simulink model "gm_pulse_detector_v4_4_vnl"  (R2017b)
settings: Solver=FixedStepDiscrete  StartTime=0.0  StopTime=SimTime  RelTol=1e-3
undefined symbols (not defined in the file or in its folder): CorrFilter, rowCorrFilter, RxSignal, threshold, WindowLen
libraries: simulink x5, dspsrcs4 x2, dsphdlfiltering x1, hdlsllib x1
settings Model: SimulationMode=accelerator  Creator=proso  LastModifiedBy=proso
settings DataIOCC: SaveOutput=off  SaveTime=off  ReturnWorkspaceOutputs=on
settings OptimizationCC: BlockReduction=off  ConditionallyExecuteInputs=off  DefaultParameterBehavior=Inlined
settings DebuggingCC: AlgebraicLoopMsg=error  InheritedTsInSrcMsg=none  SingleTaskRateTransMsg=error
settings HardwareCC: ProdBitPerPointer=32  ProdBitPerSizeT=32  ProdBitPerPtrDiffT=32  ProdLargestAtomicFloat=None  ProdIntDivRoundTo=Undefined  ProdEndianess=Unspecified  ProdWordSize=32  ProdHWDeviceType=ASIC/FPGA->ASIC/FPGA  TargetBitPerPointer=64  TargetBitPerSizeT=64  TargetBitPerPtrDiffT=64  TargetLongLongMode=on  TargetIntDivRoundTo=Zero  TargetEndianess=LittleEndian  TargetWordSize=64  TargetHWDeviceType=Custom Processor->MATLAB Host Computer  ProdEqTarget=off

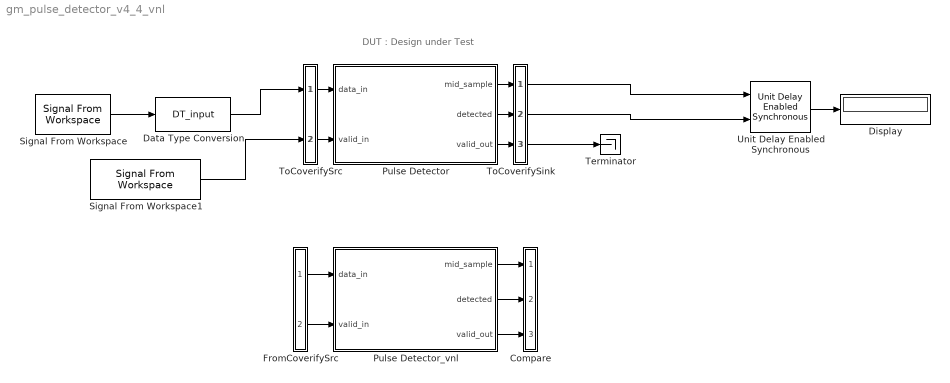
== system gm_pulse_detector_v4_4_vnl ==
  note: DUT : Design under Test
  Compare : Subsystem
      mask Display: disp('')
  Data Type Conversion : DataTypeConversion  OutDataTypeStr=DT_input
  Display : Display
  FromCoverifySrc : Subsystem
      mask Display: disp('')
  Pulse Detector : Subsystem
  Pulse Detector_vnl : Subsystem
  Signal From Workspace : dspsrcs4/Signal From Workspace  X=RxSignal  Ts=1  nsamps=1  OutputAfterFinalValue=Setting to zero  ignoreOrWarnInputAndFrameLengths=off  OutputFrames=off
  Signal From Workspace1 : dspsrcs4/Signal From Workspace  X=true(size(RxSignal))  Ts=1  nsamps=1  OutputAfterFinalValue=Setting to zero  ignoreOrWarnInputAndFrameLengths=off  OutputFrames=off
  Terminator : Terminator
  ToCoverifySink : Subsystem
      mask Display: disp('')
  ToCoverifySrc : Subsystem
      mask Display: disp('')
  Unit Delay Enabled Synchronous : hdlsllib/Discrete/Unit Delay Enabled Synchronous  InitialCondition=0.0  SampleTime=-1
      settings: SourceProductName=HDL Coder  SourceProductBaseCode=HD
  wires:
  Unit Delay Enabled Synchronous/1 -> Display/1
  Signal From Workspace/1 -> Data Type Conversion/1
  ToCoverifySrc/1(out1) -> Pulse Detector/1(data_in)
  ToCoverifySrc/2(out2) -> Pulse Detector/2(valid_in)
  Pulse Detector/1(mid_sample) -> ToCoverifySink/1(in1)
  Pulse Detector/2(detected) -> ToCoverifySink/2(in2)
  Pulse Detector/3(valid_out) -> ToCoverifySink/3(in3)
  Data Type Conversion/1 -> ToCoverifySrc/1(in1)
  Signal From Workspace1/1 -> ToCoverifySrc/2(in2)
  ToCoverifySink/1(out1) -> Unit Delay Enabled Synchronous/1
  ToCoverifySink/2(out2) -> Unit Delay Enabled Synchronous/2
  ToCoverifySink/3(out3) -> Terminator/1
  FromCoverifySrc/1(out1) -> Pulse Detector_vnl/1(data_in)
  FromCoverifySrc/2(out2) -> Pulse Detector_vnl/2(valid_in)
  Pulse Detector_vnl/1(mid_sample) -> Compare/1(in1)
  Pulse Detector_vnl/2(detected) -> Compare/2(in2)
  Pulse Detector_vnl/3(valid_out) -> Compare/3(in3)

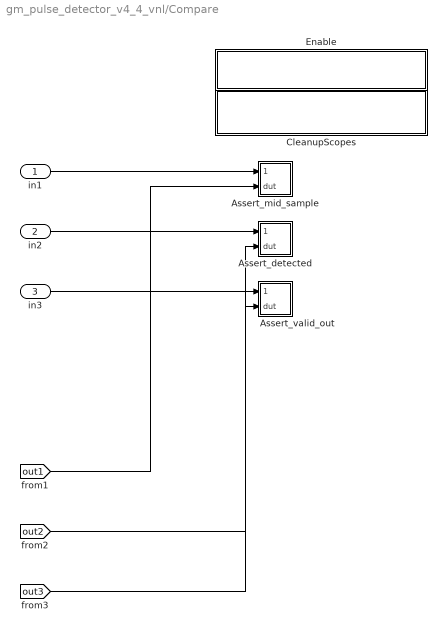
== system gm_pulse_detector_v4_4_vnl/Compare ==
  in1 : Inport
  in2 : Inport  Port=2
  in3 : Inport  Port=3
  Assert_detected : Subsystem
  Assert_mid_sample : Subsystem
  Assert_valid_out : Subsystem
  CleanupScopes : Subsystem
      settings: OpenFcn=|
      | blkName = gcb; %self block
      | idx = regexp(blkName, '/CleanupScopes$', 'once');
      | blkParent = blkName(1:idx-1);
      | blks=find_system(blkParent, 'LookUnderMasks', 'all','blocktype', 'Scope');
      | for itr = 1:length(blks)
      | 	 hScopeCfg = get_param(blks{itr},'ScopeConfiguration');
      | 	 hScopeCfg.Visible = ~ hScopeCfg.Visible;
      | end
      | drawnow;
      mask Display: fprintf(message('hdlcoder:cosim:vnl_dblclick').getString());
  Enable : Subsystem
      settings: OpenFcn=|
      | blkName = gcb;
      | idx = regexp(blkName, '/Enable$', 'once');
      | blkParent = blkName(1:idx-1);
      | blks=find_system(blkParent, 'LookUnderMasks', 'all','blocktype', 'Assertion');
      | e = get_param(blks{1}, 'Enabled');
      | if strcmp(e, 'on'), f= 'off';, else, f = 'on';, end
      | for ii=1:length(blks), set_param(blks{ii}, 'Enabled', f);, end
      | set_param(gcb, 'MaskDisplay',['fprintf(message(''hdlcoder:cosim:vnl_dblclick_assertions'',','''',upper(e),'''',').getString())']);
      mask Display: fprintf(message('hdlcoder:cosim:vnl_dblclick_assertions','OFF').getString());
  wires:
  in1/1 -> Assert_mid_sample/1(cosim)
  [out1] -> Assert_mid_sample/2(dut)
  in2/1 -> Assert_detected/1(cosim)
  [out2] -> Assert_detected/2(dut)
  in3/1 -> Assert_valid_out/1(cosim)
  [out3] -> Assert_valid_out/2(dut)

== system gm_pulse_detector_v4_4_vnl/FromCoverifySrc ==
  out1 : Outport
  out2 : Outport  Port=2
  wires:
  [in1] -> out1/1
  [in2] -> out2/1

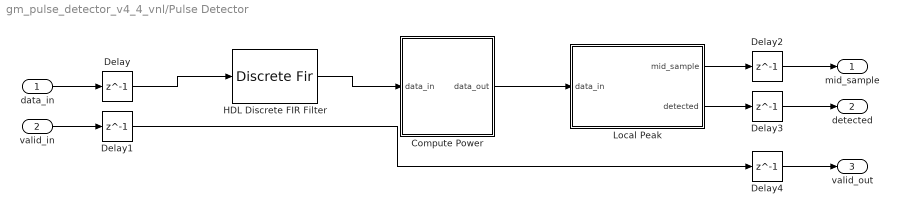
== system gm_pulse_detector_v4_4_vnl/Pulse Detector ==
  data_in : Inport  OutDataTypeStr=fixdt(1, 16, 14)  SampleTime=1
      settings: SignalType=complex
  valid_in : Inport  Port=2  OutDataTypeStr=boolean  SampleTime=1
  Compute Power : Subsystem
  Delay{,1..4} (5 alike) : Delay  DelayLength=1
  HDL Discrete FIR Filter : DiscreteFir  FilterStructure=Direct form transposed  Coefficients=CorrFilter  CoefDataTypeStr=DT_coeff
  Local Peak : Subsystem
  mid_sample : Outport
  detected : Outport  Port=2
  valid_out : Outport  Port=3
  wires:
  Local Peak/2(detected) -> Delay3/1
  Local Peak/1(mid_sample) -> Delay2/1
  HDL Discrete FIR Filter/1 -> Compute Power/1(data_in)
  Delay4/1 -> valid_out/1
  Delay3/1 -> detected/1
  Delay2/1 -> mid_sample/1
  Delay1/1 -> Delay4/1
  Delay/1 -> HDL Discrete FIR Filter/1
  Compute Power/1(data_out) -> Local Peak/1(data_in)
  valid_in/1 -> Delay1/1
  data_in/1 -> Delay/1

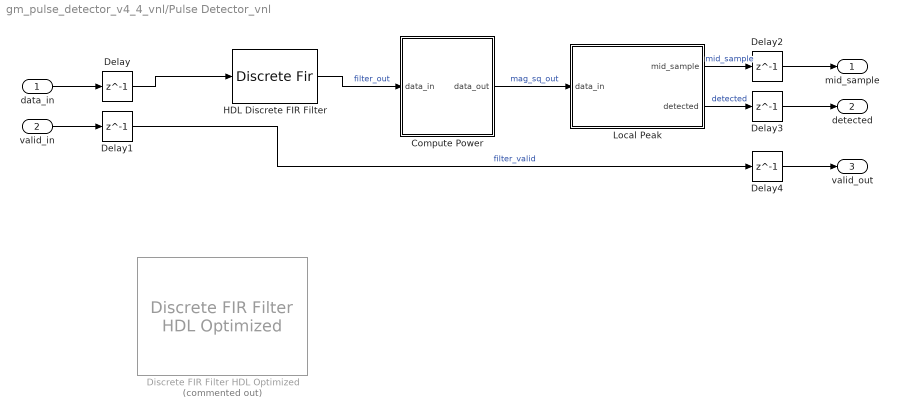
== system gm_pulse_detector_v4_4_vnl/Pulse Detector_vnl ==
  data_in : Inport
  valid_in : Inport  Port=2
  Compute Power : Subsystem
  Delay{,1..4} (5 alike) : Delay  DelayLength=1
  Discrete FIR Filter HDL Optimized : dsphdlfiltering/Discrete FIR Filter HDL Optimized  Commented=on  Numerator=real(rowCorrFilter)  Sharing=off  SharingFactor=2  SimulateUsing=Code generation  roundingMode=Floor  overflowMode=off  CoefficientsDataTypeStr=DT_coeff  CoefficientsMin=[]  CoefficientsMax=[]  OutputDataTypeStr=Inherit: Same word length as input  OutputMin=[]  OutputMax=[]  ValidInPort=on  ReadyPort=off
      settings: SourceProductName=DSP System Toolbox  SourceProductBaseCode=DS
  HDL Discrete FIR Filter : DiscreteFir  FilterStructure=Direct form transposed  Coefficients=CorrFilter  CoefDataTypeStr=DT_coeff
  Local Peak : Subsystem
  mid_sample : Outport
  detected : Outport  Port=2
  valid_out : Outport  Port=3
  wires:
  Delay4/1 -> valid_out/1
  Delay3/1 -> detected/1
  Delay2/1 -> mid_sample/1
  Delay/1 -> HDL Discrete FIR Filter/1
  Delay1/1 -> Delay4/1  "filter_valid"
  valid_in/1 -> Delay1/1
  Local Peak/2(detected) -> Delay3/1  "detected"
  data_in/1 -> Delay/1
  Local Peak/1(mid_sample) -> Delay2/1  "mid_sample"
  Compute Power/1(data_out) -> Local Peak/1(data_in)  "mag_sq_out"
  HDL Discrete FIR Filter/1 -> Compute Power/1(data_in)  "filter_out"

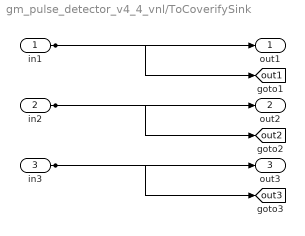
== system gm_pulse_detector_v4_4_vnl/ToCoverifySink ==
  in1 : Inport
  in2 : Inport  Port=2
  in3 : Inport  Port=3
  out1 : Outport
  out2 : Outport  Port=2
  out3 : Outport  Port=3
  tag scope: out1=global, out2=global, out3=global
  wires:
  in1/1 -> out1/1, [out1]
  in2/1 -> out2/1, [out2]
  in3/1 -> out3/1, [out3]

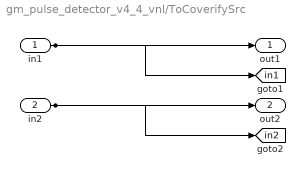
== system gm_pulse_detector_v4_4_vnl/ToCoverifySrc ==
  in1 : Inport
  in2 : Inport  Port=2
  out1 : Outport
  out2 : Outport  Port=2
  tag scope: in1=global, in2=global
  wires:
  in1/1 -> out1/1, [in1]
  in2/1 -> out2/1, [in2]

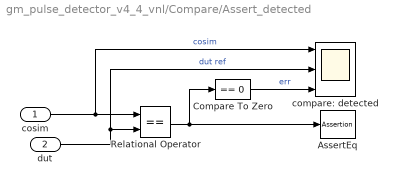
== system gm_pulse_detector_v4_4_vnl/Compare/Assert_detected ==
  cosim : Inport
  dut : Inport  Port=2
  AssertEq : Assertion  StopWhenAssertionFail=off
  Compare To Zero : simulink/Logic and Bit Operations/Compare To Zero  relop===  OutDataTypeStr=boolean
  Relational Operator : RelationalOperator  Operator===  OutDataTypeStr=boolean  RndMeth=Nearest
  compare: detected : Scope  NumInputPorts=3
  wires:
  Compare To Zero/1 -> compare: detected/3  "err"
  Relational Operator/1 -> Compare To Zero/1, AssertEq/1
  cosim/1 -> compare: detected/1, Relational Operator/1  "cosim"
  dut/1 -> compare: detected/2, Relational Operator/2  "dut ref"

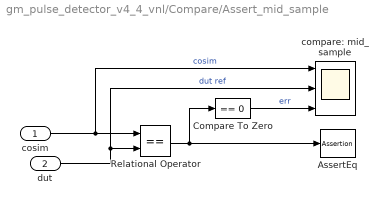
== system gm_pulse_detector_v4_4_vnl/Compare/Assert_mid_sample ==
  cosim : Inport
  dut : Inport  Port=2
  AssertEq : Assertion  StopWhenAssertionFail=off
  Compare To Zero : simulink/Logic and Bit Operations/Compare To Zero  relop===  OutDataTypeStr=boolean
  Relational Operator : RelationalOperator  Operator===  OutDataTypeStr=boolean  RndMeth=Nearest
  compare: mid_sample : Scope  NumInputPorts=3
  wires:
  Compare To Zero/1 -> compare: mid_sample/3  "err"
  Relational Operator/1 -> Compare To Zero/1, AssertEq/1
  cosim/1 -> compare: mid_sample/1, Relational Operator/1  "cosim"
  dut/1 -> compare: mid_sample/2, Relational Operator/2  "dut ref"

== system gm_pulse_detector_v4_4_vnl/Compare/Assert_valid_out ==
  cosim : Inport
  dut : Inport  Port=2
  AssertEq : Assertion  StopWhenAssertionFail=off
  Compare To Zero : simulink/Logic and Bit Operations/Compare To Zero  relop===  OutDataTypeStr=boolean
  Relational Operator : RelationalOperator  Operator===  OutDataTypeStr=boolean  RndMeth=Nearest
  compare: valid_out : Scope  NumInputPorts=3
  wires:
  Compare To Zero/1 -> compare: valid_out/3  "err"
  Relational Operator/1 -> Compare To Zero/1, AssertEq/1
  cosim/1 -> compare: valid_out/1, Relational Operator/1  "cosim"
  dut/1 -> compare: valid_out/2, Relational Operator/2  "dut ref"

== system gm_pulse_detector_v4_4_vnl/Compare/CleanupScopes ==

== system gm_pulse_detector_v4_4_vnl/Compare/Enable ==

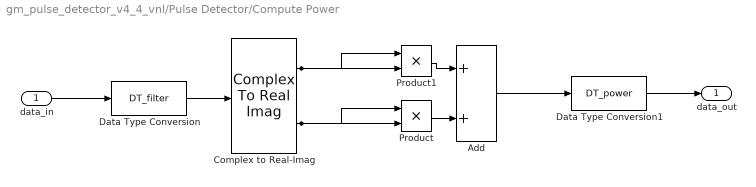
== system gm_pulse_detector_v4_4_vnl/Pulse Detector/Compute Power ==
  data_in : Inport  SampleTime=1
  Add : Sum
  Complex to Real-Imag : ComplexToRealImag
  Data Type Conversion : DataTypeConversion  OutDataTypeStr=DT_filter
  Data Type Conversion1 : DataTypeConversion  OutDataTypeStr=DT_power
  Product : Product
  Product1 : Product
  data_out : Outport
  wires:
  Product1/1 -> Add/1
  Product/1 -> Add/2
  Data Type Conversion1/1 -> data_out/1
  Data Type Conversion/1 -> Complex to Real-Imag/1
  Complex to Real-Imag/2 -> Product/1, Product/2
  Complex to Real-Imag/1 -> Product1/1, Product1/2
  Add/1 -> Data Type Conversion1/1
  data_in/1 -> Data Type Conversion/1

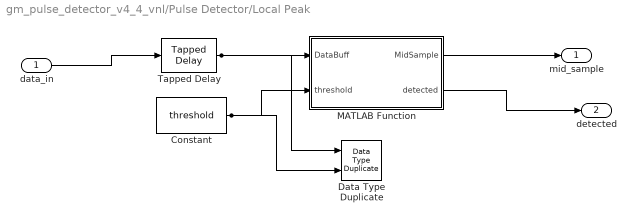
== system gm_pulse_detector_v4_4_vnl/Pulse Detector/Local Peak ==
  data_in : Inport  SampleTime=1
  Constant : Constant  Value=threshold  OutDataTypeStr=Inherit: Inherit via back propagation  SampleTime=-1
  Data Type Duplicate : DataTypeDuplicate
  MATLAB Function : Subsystem
  Tapped Delay : simulink/Discrete/Tapped Delay  vinit=0.0  samptime=-1  NumDelays=WindowLen  DelayOrder=Oldest  includeCurrent=off
  mid_sample : Outport
  detected : Outport  Port=2
  wires:
  Tapped Delay/1 -> MATLAB Function/1(DataBuff), Data Type Duplicate/1
  MATLAB Function/2(detected) -> detected/1
  MATLAB Function/1(MidSample) -> mid_sample/1
  Constant/1 -> MATLAB Function/2(threshold), Data Type Duplicate/2
  data_in/1 -> Tapped Delay/1

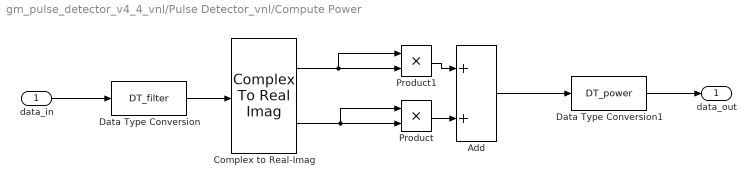
== system gm_pulse_detector_v4_4_vnl/Pulse Detector_vnl/Compute Power ==
  data_in : Inport
  Add : Sum
  Complex to Real-Imag : ComplexToRealImag
  Data Type Conversion : DataTypeConversion  OutDataTypeStr=DT_filter
  Data Type Conversion1 : DataTypeConversion  OutDataTypeStr=DT_power
  Product : Product
  Product1 : Product
  data_out : Outport
  wires:
  Data Type Conversion1/1 -> data_out/1
  Data Type Conversion/1 -> Complex to Real-Imag/1
  Complex to Real-Imag/2 -> Product/2, Product/1
  Product/1 -> Add/2
  Add/1 -> Data Type Conversion1/1
  Complex to Real-Imag/1 -> Product1/2, Product1/1
  data_in/1 -> Data Type Conversion/1
  Product1/1 -> Add/1

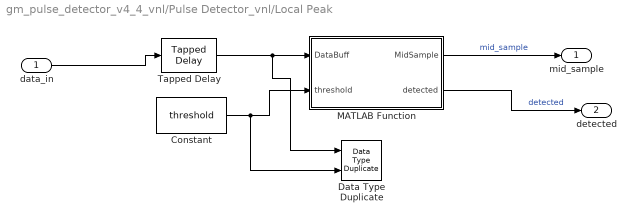
== system gm_pulse_detector_v4_4_vnl/Pulse Detector_vnl/Local Peak ==
  data_in : Inport
  Constant : Constant  Value=threshold  OutDataTypeStr=Inherit: Inherit via back propagation  SampleTime=-1
  Data Type Duplicate : DataTypeDuplicate
  MATLAB Function : MATLAB Function  TreatAsAtomicUnit=on
  Tapped Delay : simulink/Discrete/Tapped Delay  vinit=0.0  samptime=-1  NumDelays=WindowLen  DelayOrder=Oldest  includeCurrent=off
  mid_sample : Outport
  detected : Outport  Port=2
  wires:
  Constant/1 -> MATLAB Function/2(threshold), Data Type Duplicate/2
  Tapped Delay/1 -> MATLAB Function/1(DataBuff), Data Type Duplicate/1
  MATLAB Function/2(detected) -> detected/1  "detected"
  data_in/1 -> Tapped Delay/1
  MATLAB Function/1(MidSample) -> mid_sample/1  "mid_sample"

== system gm_pulse_detector_v4_4_vnl/Pulse Detector/Local Peak/MATLAB Function ==
  DataBuff : Inport  PortDimensions=11  SampleTime=1
  threshold : Inport  Port=2  SampleTime=1
  MATLAB Function : MATLAB Function  TreatAsAtomicUnit=on
  MidSample : Outport
  detected : Outport  Port=2
  wires:
  MATLAB Function/2(detected) -> detected/1
  MATLAB Function/1(MidSample) -> MidSample/1
  threshold/1 -> MATLAB Function/2(threshold)
  DataBuff/1 -> MATLAB Function/1(DataBuff)

== matlab function gm_pulse_detector_v4_4_vnl/Pulse Detector_vnl/Local Peak/MATLAB Function ==
  settings: fimath=fimath('RoundingMethod', 'Floor','OverflowAction', 'Wrap','ProductMode', 'FullPrecision', 'SumMode', 'FullPrecision')
  data: MidSample output; DataBuff input; threshold input; detected output; WindowLen parameter
function [MidSample,detected] = fcn(DataBuff,threshold, WindowLen)
   
MidIdx = ceil(WindowLen/2);
% Sliding window operation

% Compare each value in the window to the middle sample via subtraction
MidSample = DataBuff(MidIdx);
CompareOut = DataBuff - MidSample; % this is a vector

% if all values in the result are negative and the middle sample is
% greater than a threshold, it is a local max
if all(CompareOut <= 0) && (MidSample > threshold)
    detected = true;
else 
    detected = false;
end

== matlab function gm_pulse_detector_v4_4_vnl/Pulse Detector/Local Peak/MATLAB Function/MATLAB Function ==
  settings: fimath=fimath('RoundingMethod', 'Floor','OverflowAction', 'Wrap','ProductMode', 'FullPrecision', 'SumMode', 'FullPrecision')
  data: MidSample output; DataBuff input; threshold input; detected output; WindowLen parameter
function [MidSample,detected] = fcn(DataBuff,threshold, WindowLen)
   
MidIdx = ceil(WindowLen/2);
% Sliding window operation

% Compare each value in the window to the middle sample via subtraction
MidSample = DataBuff(MidIdx);
CompareOut = DataBuff - MidSample; % this is a vector

% if all values in the result are negative and the middle sample is
% greater than a threshold, it is a local max
if all(CompareOut <= 0) && (MidSample > threshold)
    detected = true;
else 
    detected = false;
end
